simulink model "Serial_debug"  (R2026a)
settings: Solver=FixedStepAuto  StopTime=inf  FixedStep=1/1000
libraries: instrumentseriallib x6, simulink x4, mcbutilslib x1
settings Model: SimulationMode=accelerator  Creator=xueji  LastModifiedBy=xuejf
settings SimscapeCC: SimscapeNominalValues="[{\"value\":\"1\",\"unit\":\"A\"},{\"value\":\"1\",\"unit\":\"bar\"},{\"value\":\"1\",\"unit\":\"cm^2\"},{\"value\":\"1\",\"unit\":\"cm^3/s\"},{\"value\":\"1\",\"unit\":\"kJ/kg\"},{\"value\":\"1\",\"unit\":\"kW\"},{\"value\":\"1\",\"unit\":\"l\"},{\"value\":\"1\",\"unit\":\"N\"},{\"value\":\"1\",\"unit\":\"N*m\"},{\"value\":\"1\",\"unit\":\"V\"}]"  SimscapeLogType=none  SimscapeLogDataHistory=5000.0

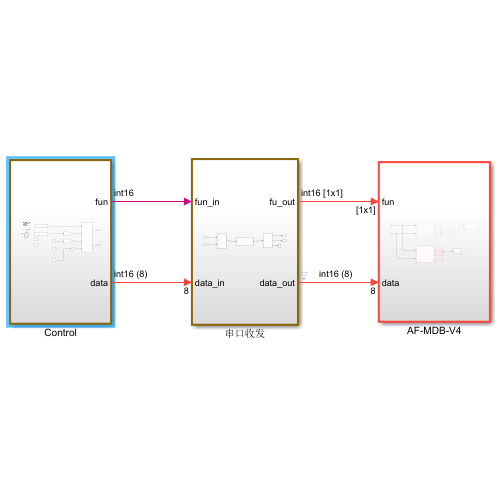
[thumbnail: Simulink's stored preview of the top-level diagram]
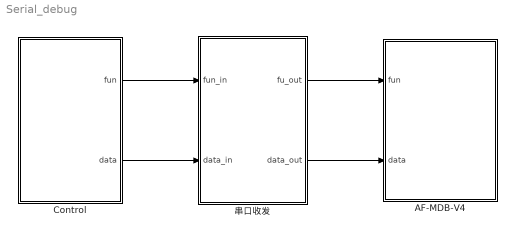
== system Serial_debug ==
  AF-MDB-V4 : Subsystem
  Control : Subsystem
  串口收发 : Subsystem
  wires:
  Control/1(fun) -> 串口收发/1(fun_in)
  Control/2(data) -> 串口收发/2(data_in)
  串口收发/1(fu_out) -> AF-MDB-V4/1(fun)
  串口收发/2(data_out) -> AF-MDB-V4/2(data)

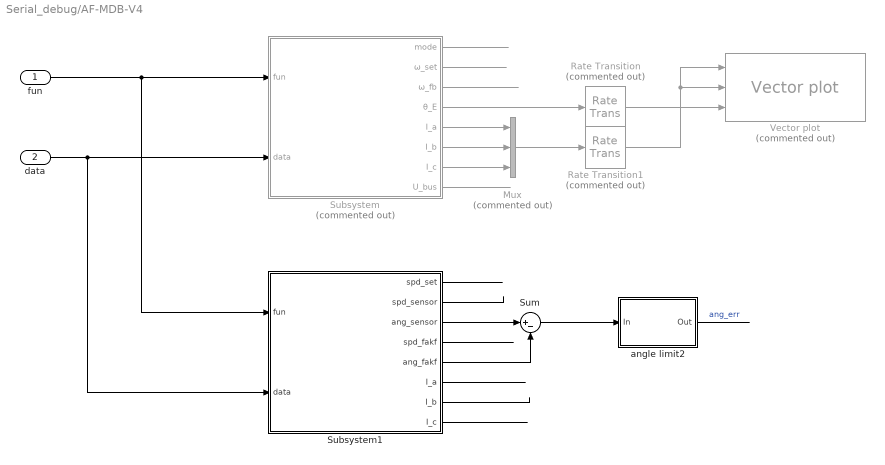
== system Serial_debug/AF-MDB-V4 ==
  fun : Inport
  data : Inport  Port=2
  Mux : Mux  Commented=on  Inputs=3
  Rate Transition : RateTransition  Commented=on  OutPortSampleTime=0.05
  Rate Transition1 : RateTransition  Commented=on  OutPortSampleTime=0.05
  Subsystem : Subsystem  Commented=on
  Subsystem1 : Subsystem
  Sum : Sum  Inputs=|+-
  Vector plot : mcbutilslib/Vector plot  Commented=on  InputSignals=Vabc Iabc Theta  ReferenceFrame=Rotating Reference Frame  axisAlign=D-axis  thetaUnits=Radians  angleUnits=Radians  OpenFigAtSimStart=on  debugEnable=0
      settings: LibrarySourceBlock=mcblib/Signal Management/Vector plot
  angle limit2 : Subsystem
  wires:
  fun/1 -> Subsystem1/1(fun), Subsystem/1(fun)
  data/1 -> Subsystem1/2(data), Subsystem/2(data)
  Subsystem/2(ω_set) -> ?
  Subsystem/3(ω_fb) -> ?
  Subsystem/4(θ_E) -> Rate Transition/1
  Subsystem/6(I_b) -> Mux/2
  Subsystem/5(I_a) -> Mux/1
  Subsystem/7(I_c) -> Mux/3
  Mux/1 -> Rate Transition1/1
  Rate Transition/1 -> Vector plot/3
  Rate Transition1/1 -> Vector plot/1, Vector plot/2
  Subsystem/8(U_bus) -> ?
  Subsystem/1(mode) -> ?
  Subsystem1/3(ang_sensor) -> Sum/1
  Subsystem1/5(ang_fakf) -> Sum/2
  Sum/1 -> angle limit2/1(In)
  angle limit2/1(Out) -> ?  "ang_err"
  Subsystem1/1(spd_set) -> ?
  Subsystem1/2(spd_sensor) -> ?
  Subsystem1/4(spd_fakf) -> ?
  Subsystem1/6(I_a) -> ?
  Subsystem1/7(I_b) -> ?
  Subsystem1/8(I_c) -> ?

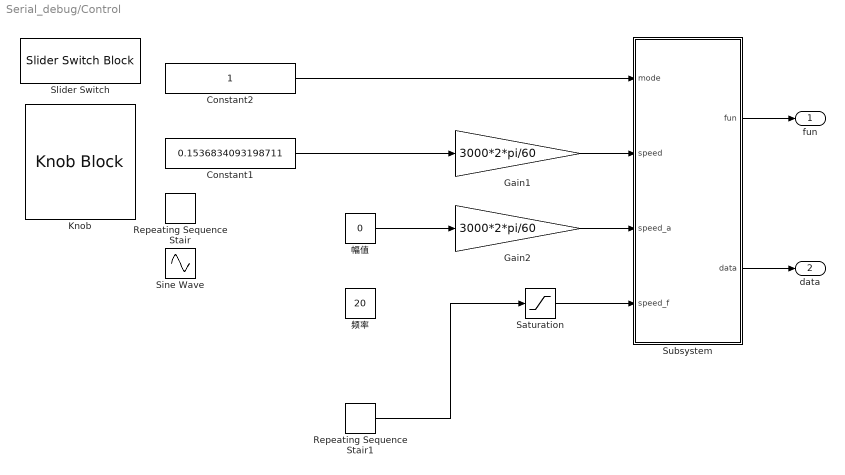
== system Serial_debug/Control ==
  Constant1 : Constant  Value=0.1536834093198711  SampleTime=-1
  Constant2 : Constant  SampleTime=0.001
  Gain1 : Gain  Gain=3000*2*pi/60
  Gain2 : Gain  Gain=3000*2*pi/60
  Knob : KnobBlock  ScaleMin=-1  ScaleMax=1  TickInterval=0.5
  Repeating Sequence Stair : simulink/Sources/Repeating Sequence Stair  OutValues=[0 0 0.05 -0.05 1 -1 0 0 0]  tsamp=1  OutMin=[]  OutMax=[]  OutDataTypeStr=double  OutputDataTypeScalingMode=double  OutDataType=fixdt(0,8)  ConRadixGroup=Best Precision: Vector-wise  OutScaling=2^-12
  Repeating Sequence Stair1 : simulink/Sources/Repeating Sequence Stair  OutValues=[0 0 5 10 20 50]  tsamp=1  OutMin=[]  OutMax=[]  OutDataTypeStr=double  OutputDataTypeScalingMode=double  OutDataType=fixdt(0,8)  ConRadixGroup=Best Precision: Vector-wise  OutScaling=2^-12
  Saturation : Saturate  UpperLimit=50  LowerLimit=0
  Sine Wave : Sin  Amplitude=0.2  Bias=0.4  Frequency=6*pi  SampleTime=0
  Slider Switch : SliderSwitchBlock
  Subsystem : Subsystem
  幅值 : Constant  Value=0
  频率 : Constant  Value=20
  fun : Outport
  data : Outport  Port=2
  wires:
  Subsystem/1(fun) -> fun/1
  Subsystem/2(data) -> data/1
  Constant2/1 -> Subsystem/1(mode)
  Constant1/1 -> Gain1/1
  Gain1/1 -> Subsystem/2(speed)
  Gain2/1 -> Subsystem/3(speed_a)
  Repeating Sequence Stair1/1 -> Saturation/1
  幅值/1 -> Gain2/1
  Saturation/1 -> Subsystem/4(speed_f)

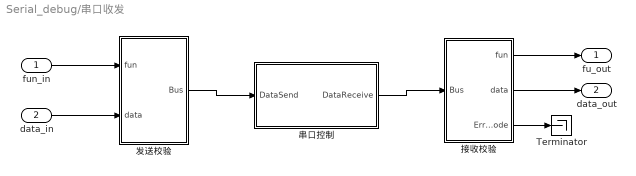
== system Serial_debug/串口收发 ==
  fun_in : Inport
  data_in : Inport  Port=2
  Terminator : Terminator
  串口控制 : Subsystem  mask{port=COM8, baud=1000000, frame_head=[0xff 0x00], frame_end=[0x00 0xff], freq_send=50, freq_rec=1000}
      mask prompts: port "端口"; baud "波特率"; frame_head "帧头"; frame_end "帧尾"; freq_send "发送频率"; freq_rec "接收频率"
      mask DialogControl DescGroupVar Prompt: 描述
      mask DialogControl DescTextVar Prompt: 串口基本参数配置，参数配置应与硬件一致，发送接收频率太快可以会卡顿或数据丢失。
      mask DialogControl ParameterGroupVar Prompt: 参数
  发送校验 : Subsystem
  接收校验 : Subsystem
  fu_out : Outport
  data_out : Outport  Port=2
  wires:
  接收校验/1(fun) -> fu_out/1
  data_in/1 -> 发送校验/2(data)
  发送校验/1(Bus) -> 串口控制/1(DataSend)
  串口控制/1(DataReceive) -> 接收校验/1(Bus)
  接收校验/2(data) -> data_out/1
  fun_in/1 -> 发送校验/1(fun)
  接收校验/3(Err_code) -> Terminator/1

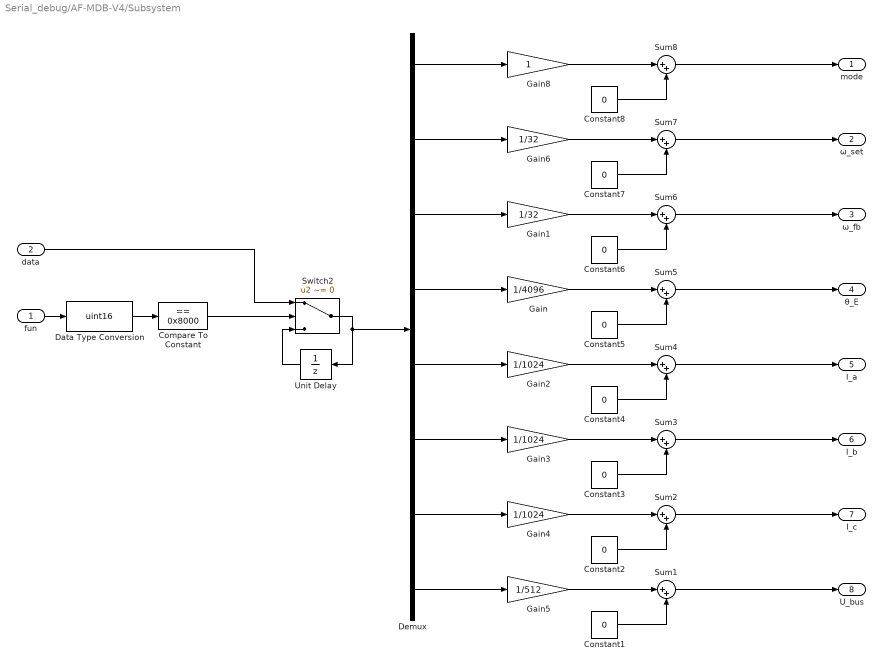
== system Serial_debug/AF-MDB-V4/Subsystem ==
  fun : Inport
  data : Inport  Port=2
  Compare To Constant : simulink/Logic and Bit Operations/Compare To Constant  relop===  const=0x8000  OutDataTypeStr=boolean
  Constant{1..8} (8 alike) : Constant  Value=0
  Data Type Conversion : DataTypeConversion  OutDataTypeStr=uint16  SaturateOnIntegerOverflow=off  RndMeth=Floor
  Demux : Demux  Outputs=8
  Gain : Gain  Gain=1/4096  OutDataTypeStr=double
  Gain1 : Gain  Gain=1/32  OutDataTypeStr=double
  Gain2 : Gain  Gain=1/1024  OutDataTypeStr=double
  Gain3 : Gain  Gain=1/1024  OutDataTypeStr=double
  Gain4 : Gain  Gain=1/1024  OutDataTypeStr=double
  Gain5 : Gain  Gain=1/512  OutDataTypeStr=double
  Gain6 : Gain  Gain=1/32  OutDataTypeStr=double
  Gain8 : Gain  OutDataTypeStr=double
  Sum{1..8} (8 alike) : Sum  Inputs=|++
  Switch2 : Switch  Criteria=u2 ~= 0  SaturateOnIntegerOverflow=off  InputSameDT=off
  Unit Delay : UnitDelay  SampleTime=-1
  mode : Outport
  ω_set : Outport  Port=2
  ω_fb : Outport  Port=3
  θ_E : Outport  Port=4
  I_a : Outport  Port=5
  I_b : Outport  Port=6
  I_c : Outport  Port=7
  U_bus : Outport  Port=8
  wires:
  Demux/8 -> Gain5/1
  Demux/5 -> Gain2/1
  Demux/3 -> Gain1/1
  Demux/7 -> Gain4/1
  Sum6/1 -> ω_fb/1
  Demux/6 -> Gain3/1
  Demux/2 -> Gain6/1
  Demux/4 -> Gain/1
  Sum1/1 -> U_bus/1
  Constant1/1 -> Sum1/2
  Gain5/1 -> Sum1/1
  Gain4/1 -> Sum2/1
  Constant2/1 -> Sum2/2
  Sum2/1 -> I_c/1
  Sum3/1 -> I_b/1
  Constant3/1 -> Sum3/2
  Gain3/1 -> Sum3/1
  Gain6/1 -> Sum7/1
  Constant7/1 -> Sum7/2
  Sum7/1 -> ω_set/1
  Constant6/1 -> Sum6/2
  Gain1/1 -> Sum6/1
  Gain/1 -> Sum5/1
  Constant5/1 -> Sum5/2
  Sum5/1 -> θ_E/1
  Sum4/1 -> I_a/1
  Constant4/1 -> Sum4/2
  Gain2/1 -> Sum4/1
  Sum8/1 -> mode/1
  Constant8/1 -> Sum8/2
  Gain8/1 -> Sum8/1
  Demux/1 -> Gain8/1
  fun/1 -> Data Type Conversion/1
  Unit Delay/1 -> Switch2/3
  Switch2/1 -> Demux/1, Unit Delay/1
  data/1 -> Switch2/1
  Compare To Constant/1 -> Switch2/2
  Data Type Conversion/1 -> Compare To Constant/1

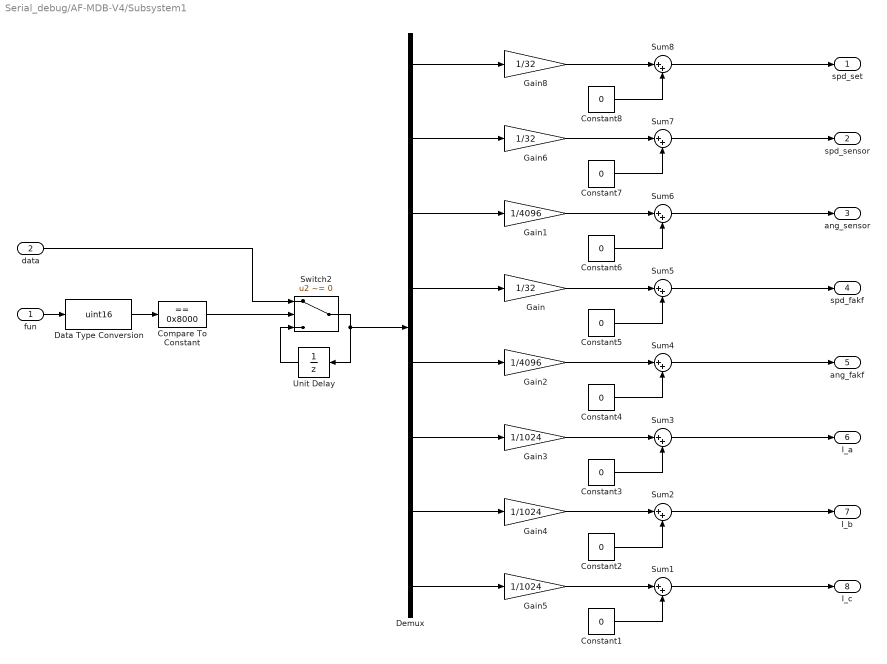
== system Serial_debug/AF-MDB-V4/Subsystem1 ==
  fun : Inport
  data : Inport  Port=2
  Compare To Constant : simulink/Logic and Bit Operations/Compare To Constant  relop===  const=0x8000  OutDataTypeStr=boolean
  Constant{1..8} (8 alike) : Constant  Value=0
  Data Type Conversion : DataTypeConversion  OutDataTypeStr=uint16  SaturateOnIntegerOverflow=off  RndMeth=Floor
  Demux : Demux  Outputs=8
  Gain : Gain  Gain=1/32  OutDataTypeStr=double
  Gain1 : Gain  Gain=1/4096  OutDataTypeStr=double
  Gain2 : Gain  Gain=1/4096  OutDataTypeStr=double
  Gain3 : Gain  Gain=1/1024  OutDataTypeStr=double
  Gain4 : Gain  Gain=1/1024  OutDataTypeStr=double
  Gain5 : Gain  Gain=1/1024  OutDataTypeStr=double
  Gain6 : Gain  Gain=1/32  OutDataTypeStr=double
  Gain8 : Gain  Gain=1/32  OutDataTypeStr=double
  Sum{1..8} (8 alike) : Sum  Inputs=|++
  Switch2 : Switch  Criteria=u2 ~= 0  SaturateOnIntegerOverflow=off  InputSameDT=off
  Unit Delay : UnitDelay  SampleTime=-1
  spd_set : Outport
  spd_sensor : Outport  Port=2
  ang_sensor : Outport  Port=3
  spd_fakf : Outport  Port=4
  ang_fakf : Outport  Port=5
  I_a : Outport  Port=6
  I_b : Outport  Port=7
  I_c : Outport  Port=8
  wires:
  Data Type Conversion/1 -> Compare To Constant/1
  Compare To Constant/1 -> Switch2/2
  data/1 -> Switch2/1
  Switch2/1 -> Unit Delay/1, Demux/1
  Unit Delay/1 -> Switch2/3
  fun/1 -> Data Type Conversion/1
  Demux/1 -> Gain8/1
  Gain8/1 -> Sum8/1
  Constant8/1 -> Sum8/2
  Sum8/1 -> spd_set/1
  Gain2/1 -> Sum4/1
  Constant4/1 -> Sum4/2
  Sum4/1 -> ang_fakf/1
  Sum5/1 -> spd_fakf/1
  Constant5/1 -> Sum5/2
  Gain/1 -> Sum5/1
  Gain1/1 -> Sum6/1
  Constant6/1 -> Sum6/2
  Sum7/1 -> spd_sensor/1
  Constant7/1 -> Sum7/2
  Gain6/1 -> Sum7/1
  Gain3/1 -> Sum3/1
  Constant3/1 -> Sum3/2
  Sum3/1 -> I_a/1
  Sum2/1 -> I_b/1
  Constant2/1 -> Sum2/2
  Gain4/1 -> Sum2/1
  Gain5/1 -> Sum1/1
  Constant1/1 -> Sum1/2
  Sum1/1 -> I_c/1
  Demux/4 -> Gain/1
  Demux/2 -> Gain6/1
  Demux/6 -> Gain3/1
  Sum6/1 -> ang_sensor/1
  Demux/7 -> Gain4/1
  Demux/3 -> Gain1/1
  Demux/5 -> Gain2/1
  Demux/8 -> Gain5/1

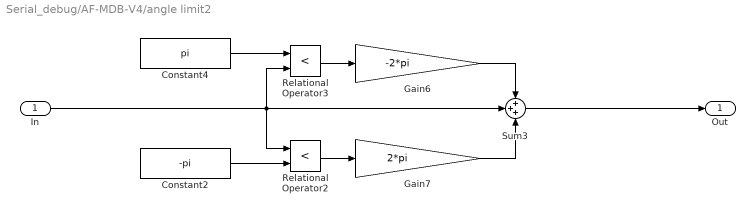
== system Serial_debug/AF-MDB-V4/angle limit2 ==
  In : Inport
  Constant2 : Constant  Value=-pi  OutDataTypeStr=single
  Constant4 : Constant  Value=pi  OutDataTypeStr=single
  Gain6 : Gain  Gain=-2*pi  OutDataTypeStr=single
  Gain7 : Gain  Gain=2*pi  OutDataTypeStr=single
  Relational Operator2 : RelationalOperator  Operator=<  RndMeth=Simplest  InputSameDT=off
  Relational Operator3 : RelationalOperator  Operator=<  RndMeth=Simplest  InputSameDT=off
  Sum3 : Sum  Inputs=+++
  Out : Outport
  wires:
  Constant2/1 -> Relational Operator2/2
  In/1 -> Relational Operator3/2, Sum3/2, Relational Operator2/1
  Constant4/1 -> Relational Operator3/1
  Relational Operator3/1 -> Gain6/1
  Gain7/1 -> Sum3/3
  Relational Operator2/1 -> Gain7/1
  Gain6/1 -> Sum3/1
  Sum3/1 -> Out/1

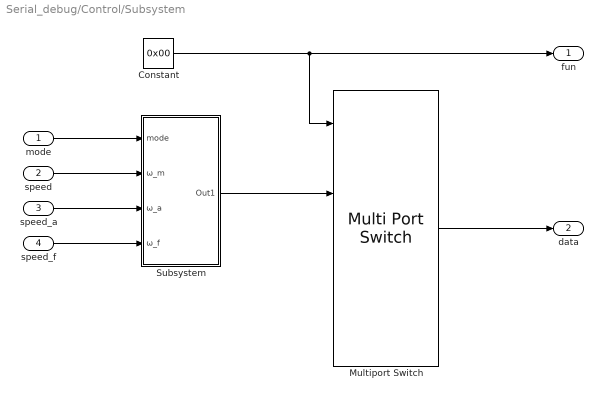
== system Serial_debug/Control/Subsystem ==
  mode : Inport
  speed : Inport  Port=2
  speed_a : Inport  Port=3
  speed_f : Inport  Port=4
  Constant : Constant  Value=0x00  OutDataTypeStr=int16
  Multiport Switch : MultiPortSwitch  DataPortOrder=Specify indices  Inputs=4  DataPortIndices={0x00 0x01}  DataPortForDefault=Additional data port  SaturateOnIntegerOverflow=off  InputSameDT=off
  Subsystem : Subsystem
  fun : Outport
  data : Outport  Port=2
  wires:
  Multiport Switch/1 -> data/1
  speed/1 -> Subsystem/2(ω_m)
  Subsystem/1(Out1) -> Multiport Switch/2
  Constant/1 -> fun/1, Multiport Switch/1
  mode/1 -> Subsystem/1(mode)
  speed_a/1 -> Subsystem/3(ω_a)
  speed_f/1 -> Subsystem/4(ω_f)

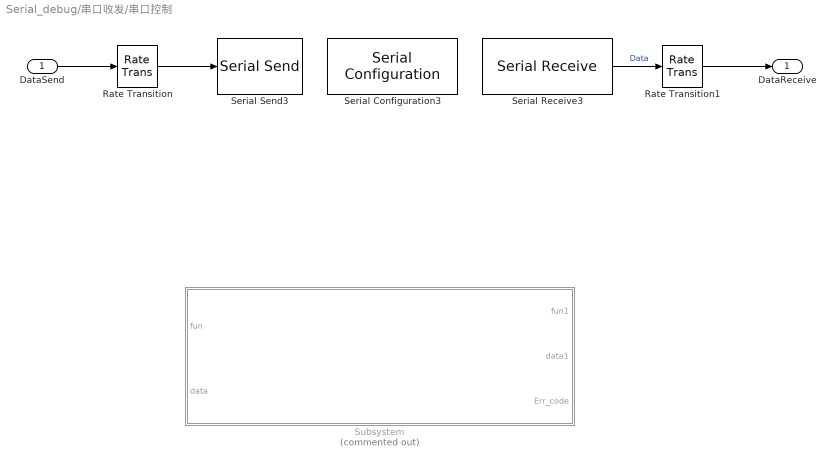
== system Serial_debug/串口收发/串口控制 ==
  DataSend : Inport
  Rate Transition : RateTransition  OutPortSampleTime=1/freq_send
  Rate Transition1 : RateTransition  OutPortSampleTime=1/freq_rec
  Serial Configuration3 : instrumentseriallib/Serial Configuration  Priority=-200000  PortSel=port  Port=port  ComPort=port  BaudRate=baud  DataBits=8  Parity=none  StopBits=1  ByteOrder=little-endian  FlowControl=none  Timeout=0.1  SimulateUsing=Interpreted execution  BlockInModel=on  aMode=1
  Serial Receive3 : instrumentseriallib/Serial Receive  Priority=1  PortSel=port  Port=port  ComPort=port  DataType=int16  SaveDataType=uint8  ToggleHeader=on  Header=frame_head  ToggleDataSize=on  DataSize=10  ToggleTerminator=on  Terminator=Custom terminator  CustomTerminator=frame_end  InputFormat=Column major  EnableBlockingMode=on  ActionDataUnavailable=Output last received value  ActionWhenDataUnavailable=Output last received value  CustomValue=0  SampleTime=-1  SimulateUsing=Interpreted execution  BlockInModel=on  aMode=1  LibraryInUse=instrumentlib
  Serial Send3 : instrumentseriallib/Serial Send  Priority=1  PortSel=port  Port=port  ComPort=port  Header=frame_head  Terminator=Custom terminator  CustomTerminator=frame_end  EnableBlockingMode=off  SimulateUsing=Interpreted execution  BlockInModel=on  aMode=1
  Subsystem : Subsystem  Commented=on
  DataReceive : Outport
  wires:
  Serial Receive3/1 -> Rate Transition1/1  "Data"
  DataSend/1 -> Rate Transition/1
  Rate Transition/1 -> Serial Send3/1
  Rate Transition1/1 -> DataReceive/1

== system Serial_debug/串口收发/发送校验 ==
  fun : Inport
  data : Inport  Port=2
  Demux2 : Demux  Outputs=8
  Matrix Sum : Sum  Inputs=+  AccumDataTypeStr=int16
  Mux : Mux  Inputs=10
  Sum : Sum  Inputs=++|
  Bus : Outport
  wires:
  Mux/1 -> Bus/1
  Demux2/1 -> Mux/2
  Demux2/3 -> Mux/4
  Demux2/5 -> Mux/6
  Demux2/7 -> Mux/8
  data/1 -> Matrix Sum/1, Demux2/1
  fun/1 -> Sum/1, Mux/1
  Demux2/2 -> Mux/3
  Demux2/4 -> Mux/5
  Demux2/6 -> Mux/7
  Demux2/8 -> Mux/9
  Matrix Sum/1 -> Sum/2
  Sum/1 -> Mux/10

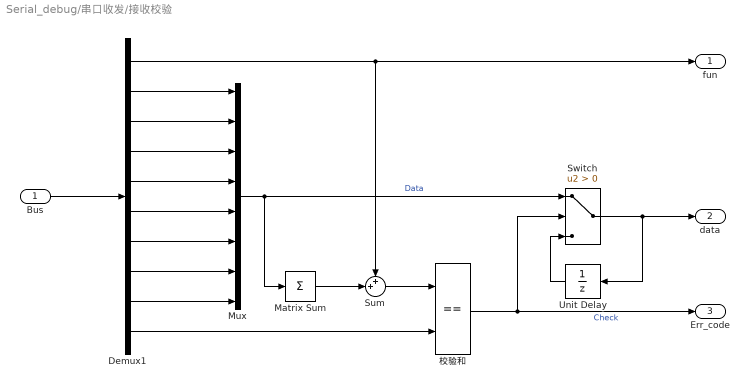
== system Serial_debug/串口收发/接收校验 ==
  Bus : Inport
  Demux1 : Demux  Outputs=10
  Matrix Sum : Sum  Inputs=+  AccumDataTypeStr=int16
  Mux : Mux  Inputs=8
  Sum : Sum  Inputs=++|
  Switch : Switch  Criteria=u2 > Threshold  SaturateOnIntegerOverflow=off  InputSameDT=off
  Unit Delay : UnitDelay  InitialCondition=[0 0 0 0 0 0 0 0]  SampleTime=-1
  校验和 : RelationalOperator  Operator===  OutDataTypeStr=boolean  RndMeth=Simplest  InputSameDT=off
  fun : Outport
  data : Outport  Port=2
  Err_code : Outport  Port=3
  wires:
  Demux1/7 -> Mux/6
  Demux1/5 -> Mux/4
  Demux1/6 -> Mux/5
  Demux1/9 -> Mux/8
  Demux1/8 -> Mux/7
  Demux1/1 -> Sum/1, fun/1
  Mux/1 -> Matrix Sum/1, Switch/1  "Data"
  Bus/1 -> Demux1/1
  Demux1/10 -> 校验和/2
  Matrix Sum/1 -> Sum/2
  校验和/1 -> Switch/2, Err_code/1  "Check"
  Switch/1 -> Unit Delay/1, data/1
  Unit Delay/1 -> Switch/3
  Demux1/2 -> Mux/1
  Demux1/3 -> Mux/2
  Demux1/4 -> Mux/3
  Sum/1 -> 校验和/1

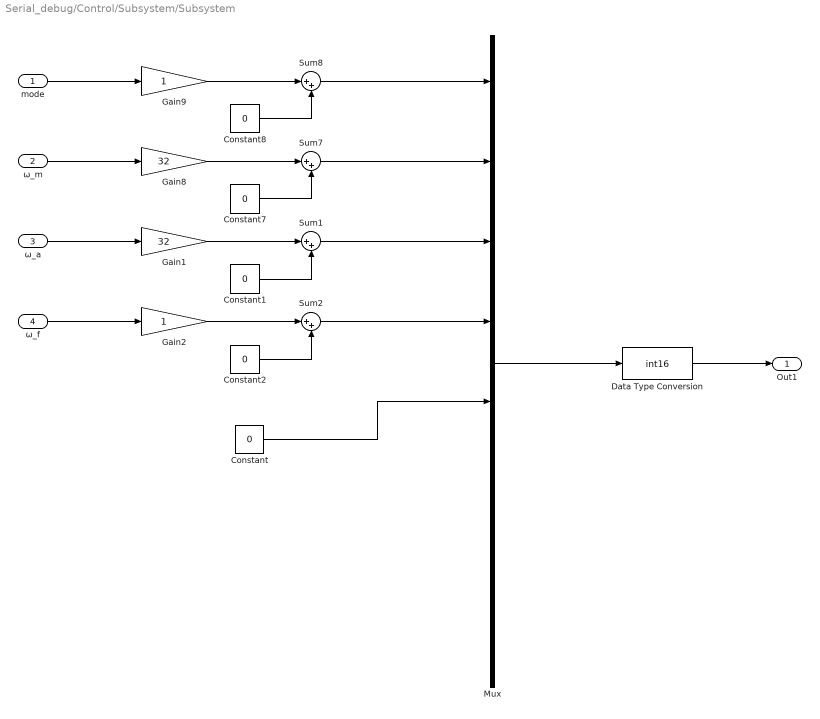
== system Serial_debug/Control/Subsystem/Subsystem ==
  mode : Inport
  ω_m : Inport  Port=2
  ω_a : Inport  Port=3
  ω_f : Inport  Port=4
  Constant{,1..2,7..8} (5 alike) : Constant  Value=0
  Data Type Conversion : DataTypeConversion  OutDataTypeStr=int16  SaturateOnIntegerOverflow=off  RndMeth=Floor
  Gain1 : Gain  Gain=32  OutDataTypeStr=double
  Gain2 : Gain  OutDataTypeStr=double
  Gain8 : Gain  Gain=32  OutDataTypeStr=double
  Gain9 : Gain  OutDataTypeStr=double
  Mux : Mux  Inputs=8
  Sum{1..2,7..8} (4 alike) : Sum  Inputs=|++
  Out1 : Outport
  wires:
  Mux/1 -> Data Type Conversion/1
  Data Type Conversion/1 -> Out1/1
  Constant7/1 -> Sum7/2
  Constant8/1 -> Sum8/2
  Sum8/1 -> Mux/1
  mode/1 -> Gain9/1
  ω_m/1 -> Gain8/1
  Gain9/1 -> Sum8/1
  Sum7/1 -> Mux/2
  Gain8/1 -> Sum7/1
  Gain1/1 -> Sum1/1
  Sum1/1 -> Mux/3
  ω_a/1 -> Gain1/1
  Constant1/1 -> Sum1/2
  Constant2/1 -> Sum2/2
  ω_f/1 -> Gain2/1
  Sum2/1 -> Mux/4
  Gain2/1 -> Sum2/1
  Constant/1 -> Mux/5

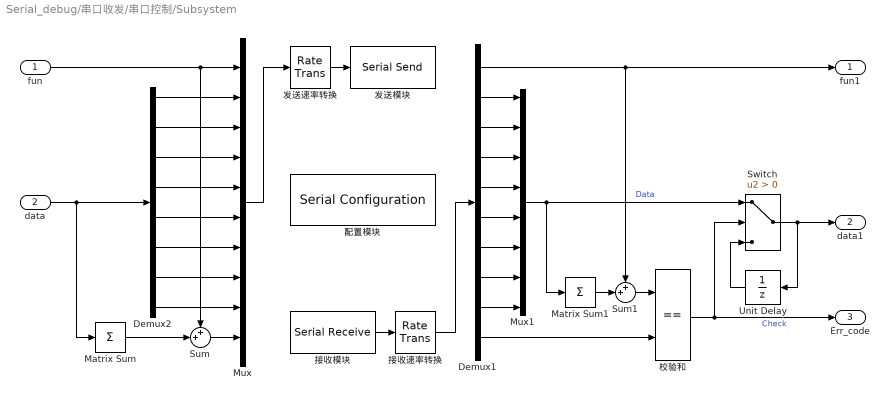
== system Serial_debug/串口收发/串口控制/Subsystem ==
  fun : Inport
  data : Inport  Port=2
  Demux1 : Demux  Outputs=10
  Demux2 : Demux  Outputs=8
  Matrix Sum : Sum  Inputs=+  AccumDataTypeStr=int16
  Matrix Sum1 : Sum  Inputs=+  AccumDataTypeStr=int16
  Mux : Mux  Inputs=10
  Mux1 : Mux  Inputs=8
  Sum : Sum  Inputs=++|
  Sum1 : Sum  Inputs=++|
  Switch : Switch  Criteria=u2 > Threshold  SaturateOnIntegerOverflow=off  InputSameDT=off
  Unit Delay : UnitDelay  InitialCondition=[0 0 0 0 0 0 0 0]  SampleTime=-1
  发送模块 : instrumentseriallib/Serial Send  Priority=1  PortSel=port  Port=port  ComPort=port  Header=frame_head  Terminator=Custom terminator  CustomTerminator=frame_end  EnableBlockingMode=off  SimulateUsing=Interpreted execution  BlockInModel=on  aMode=1
  发送速率转换 : RateTransition  OutPortSampleTime=1/freq_send
  接收模块 : instrumentseriallib/Serial Receive  Priority=1  PortSel=port  Port=port  ComPort=port  DataType=int16  SaveDataType=uint8  ToggleHeader=on  Header=frame_head  ToggleTerminator=on  Terminator=Custom terminator  CustomTerminator=frame_end  InputFormat=Column major  ToggleDataSize=on  DataSize=10  EnableBlockingMode=on  ActionDataUnavailable=Output last received value  ActionWhenDataUnavailable=Output last received value  CustomValue=0  SampleTime=-1  SimulateUsing=Interpreted execution  BlockInModel=on  aMode=1
  接收速率转换 : RateTransition  OutPortSampleTime=1/freq_rec
  校验和 : RelationalOperator  Operator===  OutDataTypeStr=boolean  RndMeth=Simplest  InputSameDT=off
  配置模块 : instrumentseriallib/Serial Configuration  Priority=-200000  PortSel=port  Port=port  ComPort=port  BaudRate=baud  DataBits=8  Parity=none  StopBits=1  ByteOrder=little-endian  FlowControl=none  Timeout=0.1  SimulateUsing=Interpreted execution  BlockInModel=on  aMode=1
  fun1 : Outport
  data1 : Outport  Port=2
  Err_code : Outport  Port=3
  wires:
  校验和/1 -> Err_code/1, Switch/2  "Check"
  Demux1/1 -> fun1/1, Sum1/1
  Demux1/2 -> Mux1/1
  Matrix Sum/1 -> Sum/2
  Demux2/2 -> Mux/3
  Demux2/3 -> Mux/4
  接收速率转换/1 -> Demux1/1
  fun/1 -> Sum/1, Mux/1
  Demux1/5 -> Mux1/4
  Demux1/7 -> Mux1/6
  Mux1/1 -> Switch/1, Matrix Sum1/1  "Data"
  Switch/1 -> data1/1, Unit Delay/1
  Demux2/6 -> Mux/7
  Demux1/10 -> 校验和/2
  Demux1/9 -> Mux1/8
  Demux2/8 -> Mux/9
  Unit Delay/1 -> Switch/3
  接收模块/1 -> 接收速率转换/1
  Demux1/8 -> Mux1/7
  Demux1/4 -> Mux1/3
  data/1 -> Matrix Sum/1, Demux2/1
  Sum1/1 -> 校验和/1
  Matrix Sum1/1 -> Sum1/2
  Sum/1 -> Mux/10
  Demux2/5 -> Mux/6
  Demux2/7 -> Mux/8
  发送速率转换/1 -> 发送模块/1
  Demux1/3 -> Mux1/2
  Demux1/6 -> Mux1/5
  Demux2/4 -> Mux/5
  Demux2/1 -> Mux/2
  Mux/1 -> 发送速率转换/1
